simulink model "Simulator_final2019"  (R2019a)
settings: Solver=ode4  StartTime=0  StopTime=500  FixedStep=0.001  RelTol=1e-3
values from neighbouring files (symbols this model uses):
  Control_Matrix = [0   Xde Xdth 0;                   0   0   0    Ydr;                   0   Zde Zdth 0;                   Lda 0   0    Ldr;                   0   Mde Mdth 0;                   Nda 0   0    Ndr]    [Autopilot_Plus_Simulator.m]
  Fg_0 = m * g * [ sin(states_0(8)) ; -cos(states_0(8))*sin(states_0(7)) ; -cos(states_0(8))*cos(states_0(7)) ]    [Autopilot_Plus_Simulator.m]
  g = aircraft_data(52)    [Autopilot_Plus_Simulator.m]
  Ixx = aircraft_data(53)    [Autopilot_Plus_Simulator.m]
  Iyy = aircraft_data(54)    [Autopilot_Plus_Simulator.m]
  Izz = aircraft_data(55)    [Autopilot_Plus_Simulator.m]
  m = aircraft_data(51)    [Autopilot_Plus_Simulator.m]
  Servo = tf(10,[1 10])    [Autopilot_Plus_Simulator.m]
  states_0 = aircraft_data(4:15)    [Autopilot_Plus_Simulator.m]
  States_Matrix = [Xu  0  Xw  0  0  0  0;                  0   Yv 0   Yp 0  Yr 0;                  Zu  0  Zw  0  Zq 0  Zwd;                  0   Lv 0   Lp 0  Lr 0;                  Mu  0  Mw  0  Mq 0  Mwd;                  0   Nv 0   Np 0  Nr 0]    [Autopilot_Plus_Simulator.m]
undefined symbols (not defined in the file or in its folder): Earth, S_0, sigbuilder_block, WGS84
libraries: simulink_extras x14, cstblocks x5, dspsigops x5, aerolibfltsims x2, aerolibtransform2 x1, shared6dof x1, aerolibasang x1, SignalEditorBlockLib x1
settings Model: Creator=Lenovo  LastModifiedBy=Elbohy

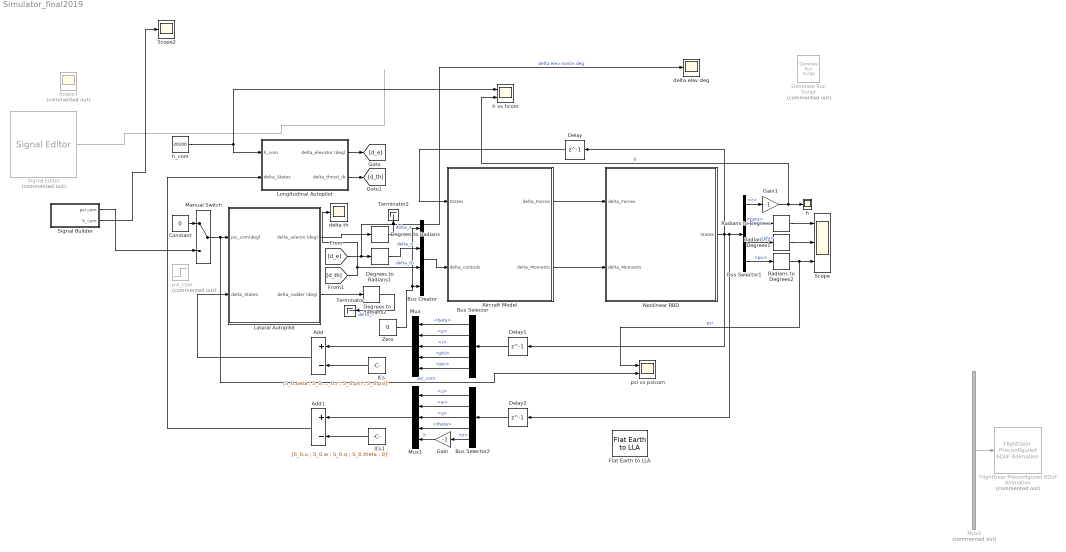
== system Simulator_final2019 ==
  Add : Sum  Inputs=+-
  Add1 : Sum  Inputs=+-
  Aircraft Model : Subsystem
  Bus Creator : BusCreator  Inputs=4
  Bus Selector : BusSelector  OutputSignals=beta,p,r,phi,psi
  Bus Selector1 : BusSelector  OutputSignals=z,beta,phi,psi
  Bus Selector2 : BusSelector  OutputSignals=u,w,q,theta,z
  Constant : Constant  Value=0
  Degrees to Radians : simulink_extras/Transformations/Degrees to Radians
  Degrees to Radians1 : simulink_extras/Transformations/Degrees to Radians
  Degrees to Radians2 : simulink_extras/Transformations/Degrees to Radians
  Delay : Delay  DelayLength=1  InitialCondition=S_0
  Delay1 : Delay  DelayLength=1  InitialCondition=S_0
  Delay2 : Delay  DelayLength=1  InitialCondition=S_0
  Flat Earth to LLA : aerolibtransform2/Flat Earth to LLA  units=Metric (MKS)  ptype=Earth (WGS84)  F=1/298.257223563  R=6378137  LL0=[0 10]  psi=0
  FlightGear Preconfigured 6DoF Animation : aerolibfltsims/FlightGear Preconfigured 6DoF Animation  Commented=on  xFlightGearVersion=v2018.2  DestinationIpAddress=127.0.0.1  DestinationPort=5502  SampleTime=1/30  packetVersion=24
      settings: SourceProductName=Aerospace Blockset
  Gain : Gain  Gain=-1
  Gain1 : Gain  Gain=-1
  Generate Run Script : aerolibfltsims/Generate Run Script  Commented=on  Architecture=Default  dataFlow=Send  GeometryModelName=HL20  AirportId=KSFO  RunwayId=10L  InitialAltitude=7224  InitialHeading=113  OffsetDistance=4.72  OffsetAzimuth=0  InstallScenery=off  DisableShaders=off  OriginAddress=127.0.0.1  DestinationPort=5502  OriginPort=5505  LocalAddress=127.0.0.1  OutputFileName=runfg.bat  FlightGearBaseDirectory=C:\Program Files\FlightGear
  ICs : Constant  Value=[S_0.beta ; S_0.p ; S_0.r ; S_0.phi ; S_0.psi]'
  ICs1 : Constant  Value=[S_0.u ; S_0.w ; S_0.q ; S_0.theta ; 0]'
  Lateral Autopilot : Subsystem
  Longitudinal Autopilot : Subsystem
  Manual Switch : ManualSwitch
  Mux : Mux  Inputs=5
  Mux1 : Mux  Inputs=5
  Mux2 : Mux  Commented=on  Inputs=6
  Nonlinear RBD : Subsystem
  Radians to Degrees : simulink_extras/Transformations/Radians to Degrees
  Radians to Degrees1 : simulink_extras/Transformations/Radians to Degrees
  Radians to Degrees2 : simulink_extras/Transformations/Radians to Degrees
  Scope : Scope  NumInputPorts=3
  Scope2 : Scope
  Scope3 : Scope  Commented=on
  Signal Builder : Subsystem  Tag=STV Subsys  LoadFcn=sigbuilder_block('load');  StartFcn=sigbuilder_block('start');  StopFcn=sigbuilder_block('stop');  ClipboardFcn=sigbuilder_block('clipboard');  mask(Sigbuilder block){tuvar=[0:10]}
      mask help: Simulink:masks:SigbuilderBlock_MD
      mask init:
      | if ~strcmp(get_param(bdroot(gcbh),'SimulationStatus'),'stopped') tuvar = sigbuilder_block('maskInit'); end
      settings: CopyFcn=sigbuilder_block('copy');  DeleteFcn=sigbuilder_block('delete');  ModelCloseFcn=sigbuilder_block('modelClose');  PreSaveFcn=sigbuilder_block('preSave');  PauseFcn=sigbuilder_block('pause');  ContinueFcn=sigbuilder_block('continue');  NameChangeFcn=sigbuilder_block('namechange');  OpenFcn=sigbuilder_block('open',[293.4 123.6 550.8 400.2 ]);  CloseFcn=sigbuilder_block('close');
      mask Display: plot(0, 0, 100, 100,[2, 2, 32, 32, 2], [68, 8, 8, 68, 68],[32, 2], [38, 38], [32, 19, 2],[53, 60, 44], [32, 17, 17, 2],[16, 16, 31, 31]);txt = getActiveGroup(gcbh);text(2, 100, txt,'verticalAlignment', 'top');
  Signal Editor : SignalEditorBlockLib/Signal Editor  Commented=on  FileName=C:\Users\amr ehab\Downloads\final task\scen.mat  ActiveScenario=Scenario  ActiveSignal=psiCommand  IsBus=off  OutputBusObjectStr=Bus: BusObject  SampleTime=0  ZeroCross=off  OutputAfterFinalValue=Holding final value  Unit=inherit  PreserveSignalName=on
      settings: SourceProductName=Simulink
  Terminator : Terminator
  Terminator2 : Terminator
  Zero : Constant  Value=0  OutDataTypeStr=Inherit: Inherit via back propagation
  "delta elav deg " : Scope
  delta th : Scope
  h : Scope
  h vs hcom : Scope  NumInputPorts=2
  h_com : Constant  Value=20100
  psi vs psicom : Scope  NumInputPorts=2
  psi_com : Step  Commented=on  After=360  SampleTime=0
  wires:
  Aircraft Model/2(delta_Moments) -> Nonlinear RBD/2(delta_Moments)
  Aircraft Model/1(delta_Forces) -> Nonlinear RBD/1(delta_Forces)
  Lateral Autopilot/1(delta_aileron (deg)) -> Degrees to Radians/1
  [d_e] -> "delta elav deg "/1, Degrees to Radians1/1  "delta elev nonlin deg"
  Lateral Autopilot/2(delta_rudder (deg)) -> Degrees to Radians2/1
  Degrees to Radians2/1 -> Terminator/1  "delta_r"
  [d_th] -> delta th/1, Bus Creator/3  "delta_th"
  Degrees to Radians1/1 -> Bus Creator/2  "delta_e"
  Degrees to Radians/1 -> Terminator2/1  "delta_a"
  Bus Creator/1 -> Aircraft Model/2(delta_controls)
  Delay/1 -> Aircraft Model/1(States)
  Delay1/1 -> Bus Selector/1
  Bus Selector/1 -> Mux/1  "<beta>"
  Bus Selector/2 -> Mux/2  "<p>"
  Bus Selector/3 -> Mux/3  "<r>"
  Bus Selector/4 -> Mux/4  "<phi>"
  Bus Selector/5 -> Mux/5  "<psi>"
  Mux/1 -> Add/1
  ICs/1 -> Add/2
  Add/1 -> Lateral Autopilot/2(delta_States)
  Bus Selector1/2 -> Radians to Degrees/1  "<beta>"
  Bus Selector1/3 -> Radians to Degrees1/1  "<phi>"
  Bus Selector1/4 -> Radians to Degrees2/1  "<psi>"
  Bus Selector1/1 -> Gain1/1  "<z>"
  Radians to Degrees/1 -> Scope/1
  Radians to Degrees2/1 -> psi vs psicom/1, Scope/3  "psi"
  Radians to Degrees1/1 -> Scope/2
  ICs1/1 -> Add1/2
  Mux1/1 -> Add1/1
  Bus Selector2/2 -> Mux1/2  "<w>"
  Bus Selector2/4 -> Mux1/4  "<theta>"
  Bus Selector2/3 -> Mux1/3  "<q>"
  Delay2/1 -> Bus Selector2/1
  Nonlinear RBD/1(States) -> Delay1/1, Delay2/1, Bus Selector1/1, Delay/1
  Bus Selector2/1 -> Mux1/1  "<u>"
  Longitudinal Autopilot/1(delta_elevator (deg)) -> [d_e]
  Longitudinal Autopilot/2("delta_thrust_ib ") -> [d_th]
  Bus Selector2/5 -> Gain/1  "<z>"
  Add1/1 -> Longitudinal Autopilot/2(delta_States)
  Gain/1 -> Mux1/5  "h"
  Manual Switch/1 -> psi vs psicom/2, Lateral Autopilot/1(psi_com(deg))  "psi_com"
  Constant/1 -> Manual Switch/1
  Gain1/1 -> h vs hcom/2, h/1  "h"
  ? -> Scope3/1
  Signal Editor/1 -> ?
  Mux2/1 -> FlightGear Preconfigured 6DoF Animation/1
  ? -> Mux2/1
  ? -> Mux2/2
  ? -> Mux2/3
  ? -> Mux2/4
  ? -> Mux2/5
  ? -> Mux2/6
  Signal Builder/2(h_com) -> Scope2/1
  Signal Builder/1(psi com) -> Manual Switch/2
  h_com/1 -> Longitudinal Autopilot/1(h_com), h vs hcom/1
  Zero/1 -> Bus Creator/1, Bus Creator/4

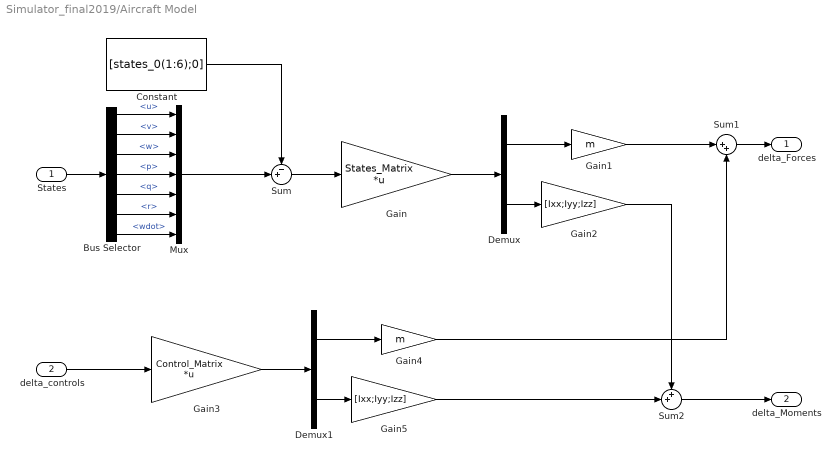
== system Simulator_final2019/Aircraft Model ==
  States : Inport
  delta_controls : Inport  Port=2
  Bus Selector : BusSelector  OutputSignals=u,v,w,p,q,r,wdot
  Constant : Constant  Value=[states_0(1:6);0]
  Demux : Demux  Outputs=2
  Demux1 : Demux  Outputs=2
  Gain : Gain  Gain=States_Matrix  Multiplication=Matrix(K*u)
  Gain1 : Gain  Gain=m
  Gain2 : Gain  Gain=[Ixx;Iyy;Izz]
  Gain3 : Gain  Gain=Control_Matrix  Multiplication=Matrix(K*u)
  Gain4 : Gain  Gain=m
  Gain5 : Gain  Gain=[Ixx;Iyy;Izz]
  Mux : Mux  Inputs=7
  Sum : Sum  Inputs=-+|
  Sum1 : Sum  Inputs=|++
  Sum2 : Sum  Inputs=++|
  delta_Forces : Outport  VectorParamsAs1DForOutWhenUnconnected=on
  delta_Moments : Outport  Port=2  VectorParamsAs1DForOutWhenUnconnected=on
  wires:
  Gain5/1 -> Sum2/2
  Gain1/1 -> Sum1/1
  Demux/2 -> Gain2/1
  Constant/1 -> Sum/1
  Gain/1 -> Demux/1
  Sum/1 -> Gain/1
  Mux/1 -> Sum/2
  Gain3/1 -> Demux1/1
  Gain4/1 -> Sum1/2
  Demux/1 -> Gain1/1
  Demux1/1 -> Gain4/1
  Demux1/2 -> Gain5/1
  Gain2/1 -> Sum2/1
  Sum1/1 -> delta_Forces/1
  Sum2/1 -> delta_Moments/1
  Bus Selector/1 -> Mux/1  "<u>"
  Bus Selector/2 -> Mux/2  "<v>"
  Bus Selector/3 -> Mux/3  "<w>"
  Bus Selector/4 -> Mux/4  "<p>"
  Bus Selector/5 -> Mux/5  "<q>"
  Bus Selector/6 -> Mux/6  "<r>"
  Bus Selector/7 -> Mux/7  "<wdot>"
  States/1 -> Bus Selector/1
  delta_controls/1 -> Gain3/1

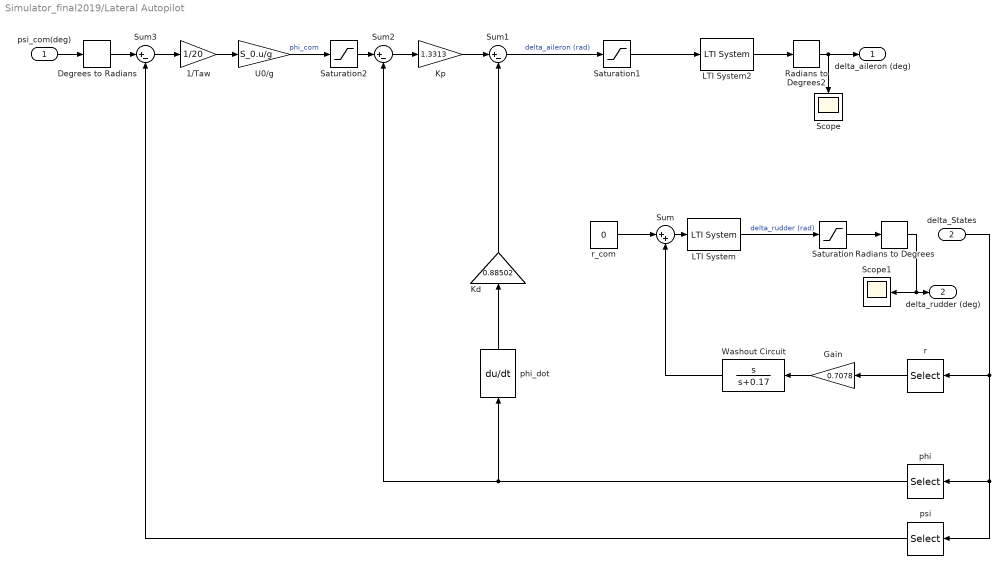
== system Simulator_final2019/Lateral Autopilot ==
  psi_com(deg) : Inport
  delta_States : Inport  Port=2
  1/Taw : Gain  Gain=1/20
  Degrees to Radians : simulink_extras/Transformations/Degrees to Radians
  Gain : Gain  Gain=0.7078
  Kd : Gain  Gain=0.88502
  Kp : Gain  Gain=1.3313
  LTI System : cstblocks/LTI System  sys=servo  IC=[]
  LTI System2 : cstblocks/LTI System  sys=servo  IC=[]
  Radians to Degrees : simulink_extras/Transformations/Radians to Degrees
  Radians to Degrees2 : simulink_extras/Transformations/Radians to Degrees
  Saturation : Saturate  UpperLimit=15*pi/180  LowerLimit=-15*pi/180
  Saturation1 : Saturate  UpperLimit=50*pi/180  LowerLimit=-50*pi/180
  Saturation2 : Saturate  UpperLimit=30*pi/180  LowerLimit=-30*pi/180
  Scope : Scope
  Scope1 : Scope
  Sum : Sum  Inputs=|++
  Sum1 : Sum  Inputs=|+-
  Sum2 : Sum  Inputs=|+-
  Sum3 : Sum  Inputs=|+-
  U0/g : Gain  Gain=S_0.u/g
  Washout Circuit : TransferFcn  Numerator=[1 0]  Denominator=[1 0.17]
  phi : Selector  InputPortWidth=5  IndexOptions=Index vector (dialog)  Indices=[4]  OutputSizes=1
  phi_dot : Derivative
  psi : Selector  InputPortWidth=5  IndexOptions=Index vector (dialog)  Indices=[5]  OutputSizes=1
  r : Selector  InputPortWidth=5  IndexOptions=Index vector (dialog)  Indices=[3]  OutputSizes=1
  r_com : Constant  Value=0
  delta_aileron (deg) : Outport  VectorParamsAs1DForOutWhenUnconnected=on
  delta_rudder (deg) : Outport  Port=2  VectorParamsAs1DForOutWhenUnconnected=on
  wires:
  LTI System2/1 -> Radians to Degrees2/1
  1/Taw/1 -> U0/g/1
  Kp/1 -> Sum1/1
  Radians to Degrees2/1 -> delta_aileron (deg)/1, Scope/1
  Sum1/1 -> Saturation1/1  "delta_aileron (rad)"
  delta_States/1 -> phi/1, psi/1, r/1
  Saturation2/1 -> Sum2/1
  Radians to Degrees/1 -> Scope1/1, delta_rudder (deg)/1
  Kd/1 -> Sum1/2
  Sum2/1 -> Kp/1
  psi/1 -> Sum3/2
  Saturation1/1 -> LTI System2/1
  LTI System/1 -> Saturation/1  "delta_rudder (rad)"
  phi/1 -> Sum2/2, phi_dot/1
  Gain/1 -> Washout Circuit/1
  Sum3/1 -> 1/Taw/1
  Washout Circuit/1 -> Sum/2
  r_com/1 -> Sum/1
  r/1 -> Gain/1
  Degrees to Radians/1 -> Sum3/1
  U0/g/1 -> Saturation2/1  "phi_com"
  Saturation/1 -> Radians to Degrees/1
  phi_dot/1 -> Kd/1
  Sum/1 -> LTI System/1
  psi_com(deg)/1 -> Degrees to Radians/1

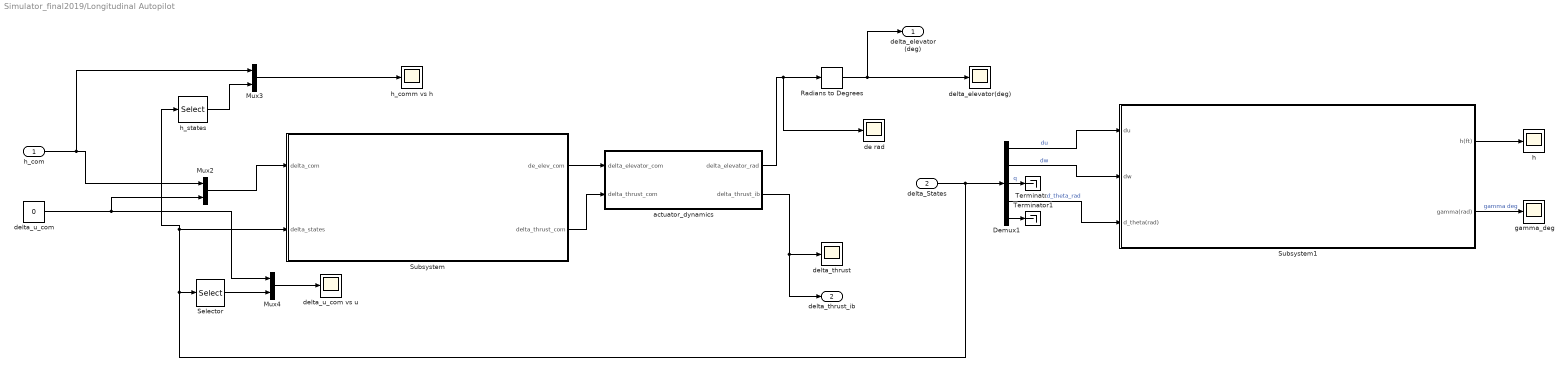
== system Simulator_final2019/Longitudinal Autopilot ==
  h_com : Inport
  delta_States : Inport  Port=2
  Demux1 : Demux  Outputs=5
  Mux2 : Mux  Inputs=2
  Mux3 : Mux  Inputs=2
  Mux4 : Mux  Inputs=2
  Radians to Degrees : simulink_extras/Transformations/Radians to Degrees
  Selector : Selector  InputPortWidth=5  IndexOptions=Index vector (dialog)  Indices=[1]  OutputSizes=1
  Subsystem : Subsystem
  Subsystem1 : Subsystem
  Terminator : Terminator
  Terminator1 : Terminator
  "actuator_dynamics " : Subsystem
  de rad : Scope
  delta_elevator(deg) : Scope
  delta_thrust : Scope
  delta_u_com : Constant  Value=0
  "delta_u_com vs u " : Scope
  gamma_deg : Scope
  h : Scope
  h_comm vs h : Scope
  h_states : Selector  InputPortWidth=5  IndexOptions=Index vector (dialog)  Indices=[5]  OutputSizes=1
  delta_elevator (deg) : Outport  VectorParamsAs1DForOutWhenUnconnected=on
  "delta_thrust_ib " : Outport  Port=2  VectorParamsAs1DForOutWhenUnconnected=on
  wires:
  h_com/1 -> Mux3/1, Mux2/1
  Mux2/1 -> Subsystem/1(delta_com)
  Radians to Degrees/1 -> delta_elevator (deg)/1, delta_elevator(deg)/1
  Subsystem1/1("h(ft) ") -> h/1
  Subsystem/2(delta_thrust_com) -> "actuator_dynamics "/2("delta_thrust_com ")
  delta_States/1 -> Selector/1, h_states/1, Subsystem/2("delta_states "), Demux1/1
  delta_u_com/1 -> Mux4/1, Mux2/2
  Selector/1 -> Mux4/2
  Demux1/1 -> Subsystem1/1("du ")  "du"
  Subsystem1/2(gamma(rad)) -> gamma_deg/1  "gamma deg"
  Demux1/4 -> Subsystem1/3(d_theta(rad))  "d_theta_rad"
  "actuator_dynamics "/2("delta_thrust_ib ") -> "delta_thrust_ib "/1, delta_thrust/1
  h_states/1 -> Mux3/2
  Demux1/2 -> Subsystem1/2(dw)  "dw"
  Mux3/1 -> h_comm vs h/1
  "actuator_dynamics "/1(delta_elevator_rad) -> de rad/1, Radians to Degrees/1
  Subsystem/1(de_elev_com) -> "actuator_dynamics "/1("delta_elevator_com ")
  Mux4/1 -> "delta_u_com vs u "/1
  Demux1/3 -> Terminator/1  "q"
  Demux1/5 -> Terminator1/1

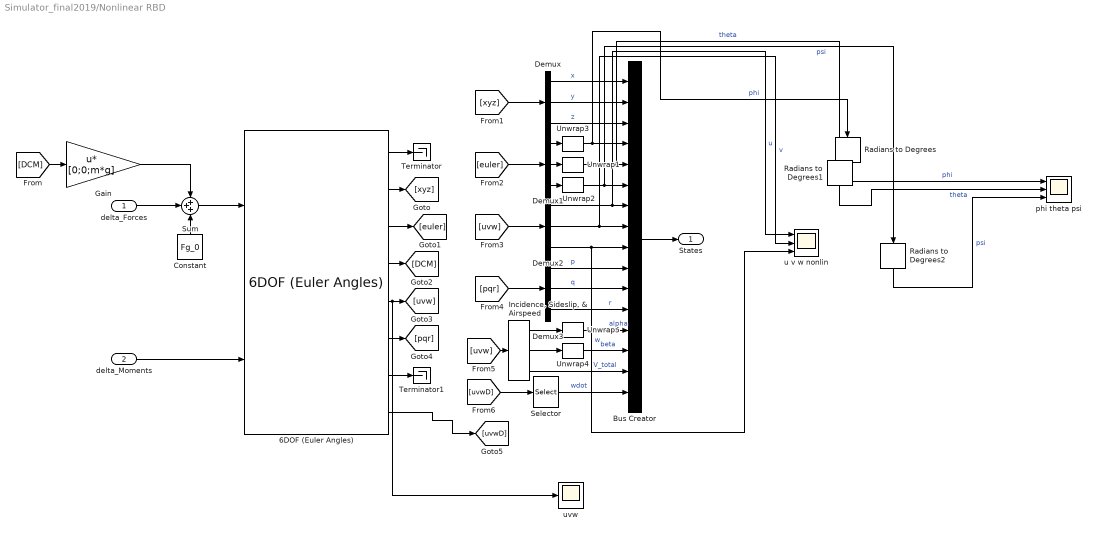
== system Simulator_final2019/Nonlinear RBD ==
  delta_Forces : Inport
  delta_Moments : Inport  Port=2
  6DOF (Euler Angles) : shared6dof/6DOF (Euler Angles)  units=English (Velocity in ft/s)  mtype=Fixed  rep=Euler Angles  xme_0=states_0(10:12)  Vm_0=states_0(1:3)  eul_0=states_0(7:9)  pm_0=states_0(4:6)  mass_0=m  mass_e=0.5  mass_f=2.0  inertia=I  inertia_e=eye(3)  inertia_f=2*eye(3)  k_quat=1.0  vre_flag=on  abi_flag=off  aMode=0  xme_statename=''  Vm_statename=''  eul_statename=''  quat_statename=''  pm_statename=''  mass_statename=''
      settings: SourceProductBaseCode=AE
  Bus Creator : BusCreator  Inputs=16
  Constant : Constant  Value=Fg_0
  Demux{,1..3} (4 alike) : Demux  Outputs=3
  Gain : Gain  Gain=[0;0;m*g]  Multiplication=Matrix(u*K)
  "Incidence, Sideslip, & Airspeed" : aerolibasang/Incidence, Sideslip, & Airspeed
      settings: SourceProductName=Aerospace Blockset
  Radians to Degrees : simulink_extras/Transformations/Radians to Degrees
  Radians to Degrees1 : simulink_extras/Transformations/Radians to Degrees
  Radians to Degrees2 : simulink_extras/Transformations/Radians to Degrees
  Selector : Selector  InputPortWidth=3  IndexOptions=Index vector (dialog)  Indices=[3]  OutputSizes=1
  Sum : Sum  Inputs=+++
  Terminator : Terminator
  Terminator1 : Terminator
  Unwrap{1..5} (5 alike) : dspsigops/Unwrap  tol=pi  InputProcessing=Columns as channels (frame based)  running=off
  phi theta psi : Scope  NumInputPorts=3
  u v w nonlin : Scope  NumInputPorts=3
  "uvw " : Scope
  States : Outport  VectorParamsAs1DForOutWhenUnconnected=on
  wires:
  Demux2/1 -> u v w nonlin/1, Bus Creator/7  "u"
  Selector/1 -> Bus Creator/16  "wdot"
  Demux/1 -> Bus Creator/1  "x"
  Demux1/1 -> Unwrap3/1
  Demux3/3 -> Bus Creator/12  "r"
  Demux3/2 -> Bus Creator/11  "q"
  [xyz] -> Demux/1
  Demux1/2 -> Unwrap1/1
  Demux/3 -> Bus Creator/3  "z"
  [pqr] -> Demux3/1
  [uvw] -> Demux2/1
  [uvw] -> "Incidence, Sideslip, & Airspeed"/1
  Gain/1 -> Sum/1
  6DOF (Euler Angles)/5 -> "uvw "/1, [uvw]
  "Incidence, Sideslip, & Airspeed"/3 -> Bus Creator/15  "V_total"
  6DOF (Euler Angles)/3 -> [euler]
  6DOF (Euler Angles)/4 -> [DCM]
  Demux2/2 -> u v w nonlin/2, Bus Creator/8  "v"
  Demux2/3 -> u v w nonlin/3, Bus Creator/9  "w"
  6DOF (Euler Angles)/6 -> [pqr]
  Demux/2 -> Bus Creator/2  "y"
  [uvwD] -> Selector/1
  6DOF (Euler Angles)/1 -> Terminator/1
  Sum/1 -> 6DOF (Euler Angles)/1
  6DOF (Euler Angles)/8 -> [uvwD]
  [euler] -> Demux1/1
  [DCM] -> Gain/1
  6DOF (Euler Angles)/7 -> Terminator1/1
  Demux3/1 -> Bus Creator/10  "p"
  Constant/1 -> Sum/3
  6DOF (Euler Angles)/2 -> [xyz]
  delta_Forces/1 -> Sum/2
  delta_Moments/1 -> 6DOF (Euler Angles)/2
  Bus Creator/1 -> States/1
  Unwrap1/1 -> Radians to Degrees1/1, Bus Creator/5  "theta"
  Demux1/3 -> Unwrap2/1
  Unwrap3/1 -> Radians to Degrees/1, Bus Creator/4  "phi"
  Unwrap2/1 -> Bus Creator/6, Radians to Degrees2/1  "psi"
  "Incidence, Sideslip, & Airspeed"/2 -> Unwrap4/1
  Unwrap5/1 -> Bus Creator/13  "alpha"
  Unwrap4/1 -> Bus Creator/14  "beta"
  "Incidence, Sideslip, & Airspeed"/1 -> Unwrap5/1
  Radians to Degrees/1 -> phi theta psi/1  "phi"
  Radians to Degrees1/1 -> phi theta psi/2  "theta"
  Radians to Degrees2/1 -> phi theta psi/3  "psi"

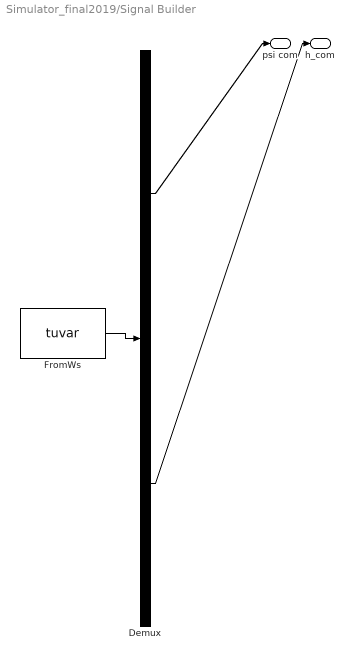
== system Simulator_final2019/Signal Builder ==
  Demux : Demux  Tag=STV Demux  Outputs=2
  FromWs : FromWorkspace  Tag=STV FromWs  VariableName=tuvar  SampleTime=0
      SigBuilderData=|
      | common.afterFinalStr = 'Extrapolate'
      | common.sampleTime = 0
      | dataSet.timeRange = [0 1800]
      | dataSet.name = 'Group 1'
      | sbobj.Groups.Name = 'Group 1'
      | sbobj.Groups.Signals(1).Name = 'psi com'
      | sbobj.Groups.Signals(1).XData = [0 720 720 1080 1080 1800]
      | sbobj.Groups.Signals(1).YData = [0 0 360 360 390 390]
      | sbobj.Groups.Signals(2).Name = 'h_com'
      | sbobj.Groups.Signals(2).XData = [0 600 1080 1080 1200 1800]
      | sbobj.Groups.Signals(2).YData = [20000 30000 30000 30100 30100 20000]
      | sbobj.Groups.TimeRange = [0 1800]
  psi com : Outport  Tag=STV Outport
  h_com : Outport  Tag=STV Outport  Port=2
  wires:
  FromWs/1 -> Demux/1
  Demux/1 -> psi com/1
  Demux/2 -> h_com/1

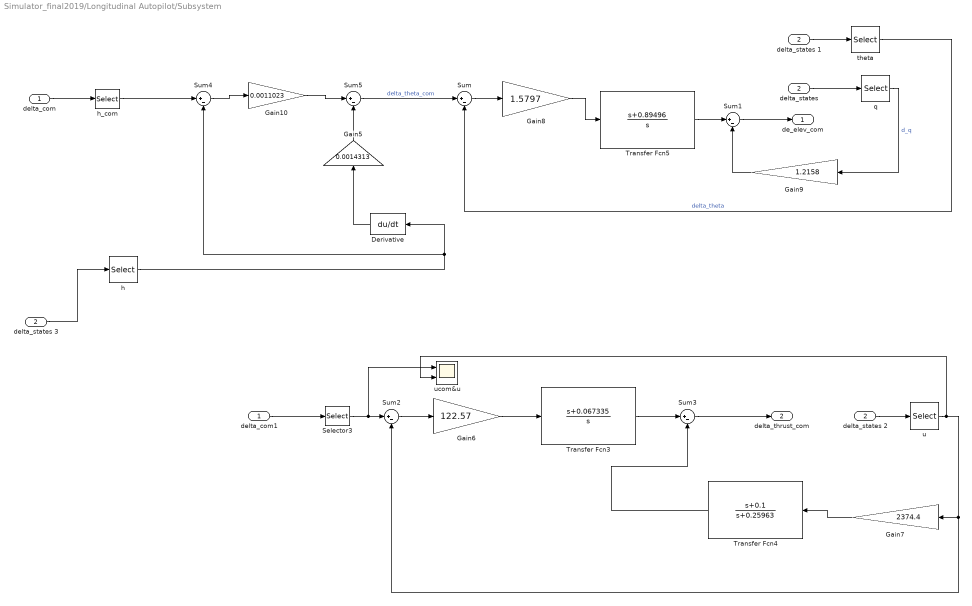
== system Simulator_final2019/Longitudinal Autopilot/Subsystem ==
  delta_com : Inport
  "delta_states " : Inport  Port=2
  Derivative : Derivative
  Gain10 : Gain  Gain=0.0011023
  Gain5 : Gain  Gain=0.0014313
  Gain6 : Gain  Gain=122.57
  Gain7 : Gain  Gain=2374.4
  Gain8 : Gain  Gain=1.5797
  Gain9 : Gain  Gain=1.2158
  Selector3 : Selector  InputPortWidth=2  IndexOptions=Index vector (dialog)  Indices=[2]  OutputSizes=1
  Sum{,1..5} (6 alike) : Sum  Inputs=|+-
  Transfer Fcn3 : TransferFcn  Numerator=[1 0.067335]  Denominator=[1 0]
  Transfer Fcn4 : TransferFcn  Numerator=[1 0.1]  Denominator=[1 0.25963]
  Transfer Fcn5 : TransferFcn  Numerator=[1 0.89496]  Denominator=[1 0]
  delta_com1 : InportShadow
  delta_states 1 : InportShadow  Port=2
  delta_states 2 : InportShadow  Port=2
  delta_states 3 : InportShadow  Port=2
  h : Selector  InputPortWidth=5  IndexOptions=Index vector (dialog)  Indices=[5]  OutputSizes=1
  h_com : Selector  InputPortWidth=2  IndexOptions=Index vector (dialog)  Indices=[1]  OutputSizes=1
  "q " : Selector  InputPortWidth=5  IndexOptions=Index vector (dialog)  Indices=[3]  OutputSizes=1
  "theta " : Selector  InputPortWidth=5  IndexOptions=Index vector (dialog)  Indices=[4]  OutputSizes=1
  u : Selector  InputPortWidth=5  IndexOptions=Index vector (dialog)  Indices=[1]  OutputSizes=1
  ucom&u : Scope  NumInputPorts=2
  de_elev_com : Outport
  delta_thrust_com : Outport  Port=2
  wires:
  Gain10/1 -> Sum5/1
  Gain5/1 -> Sum5/2
  Gain8/1 -> Transfer Fcn5/1
  delta_com/1 -> h_com/1
  Sum/1 -> Gain8/1
  delta_states 3/1 -> h/1
  h/1 -> Derivative/1, Sum4/2
  delta_com1/1 -> Selector3/1
  delta_states 2/1 -> u/1
  Gain7/1 -> Transfer Fcn4/1
  "delta_states "/1 -> "q "/1
  "q "/1 -> Gain9/1  "d_q"
  delta_states 1/1 -> "theta "/1
  Gain6/1 -> Transfer Fcn3/1
  Sum1/1 -> de_elev_com/1
  Transfer Fcn4/1 -> Sum3/2
  Transfer Fcn5/1 -> Sum1/1
  Sum5/1 -> Sum/1  "delta_theta_com"
  Selector3/1 -> ucom&u/1, Sum2/1
  Gain9/1 -> Sum1/2
  Sum4/1 -> Gain10/1
  "theta "/1 -> Sum/2  "delta_theta"
  Transfer Fcn3/1 -> Sum3/1
  u/1 -> ucom&u/2, Gain7/1, Sum2/2
  Sum2/1 -> Gain6/1
  h_com/1 -> Sum4/1
  Sum3/1 -> delta_thrust_com/1
  Derivative/1 -> Gain5/1

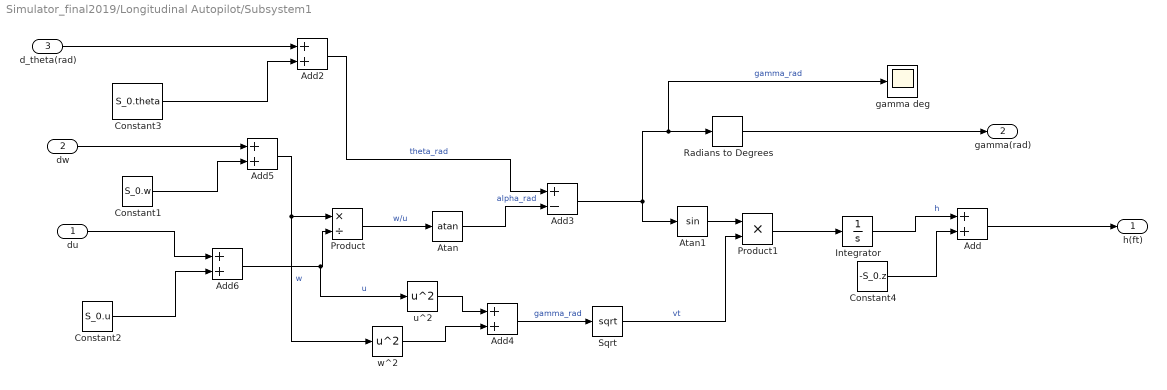
== system Simulator_final2019/Longitudinal Autopilot/Subsystem1 ==
  "du " : Inport
  dw : Inport  Port=2
  d_theta(rad) : Inport  Port=3
  Add{,2,4..6} (5 alike) : Sum
  Add3 : Sum  Inputs=+-
  Atan : Trigonometry  Operator=atan
  Atan1 : Trigonometry
  Constant1 : Constant  Value=S_0.w
  Constant2 : Constant  Value=S_0.u
  Constant3 : Constant  Value=S_0.theta
  Constant4 : Constant  Value=-S_0.z
  Integrator : Integrator
  Product : Product  Inputs=*/
  Product1 : Product
  Radians to Degrees : simulink_extras/Transformations/Radians to Degrees
  Sqrt : Sqrt  SaturateOnIntegerOverflow=on
  gamma deg : Scope
  u^2 : Math  Operator=square  SaturateOnIntegerOverflow=on
  w^2 : Math  Operator=square  SaturateOnIntegerOverflow=on
  "h(ft) " : Outport
  gamma(rad) : Outport  Port=2
  wires:
  Product1/1 -> Integrator/1
  Constant4/1 -> Add/2
  Radians to Degrees/1 -> gamma(rad)/1
  Integrator/1 -> Add/1  "h"
  dw/1 -> Add5/1
  d_theta(rad)/1 -> Add2/1
  Atan/1 -> Add3/2  "alpha_rad"
  Constant2/1 -> Add6/2
  Constant1/1 -> Add5/2
  Add4/1 -> Sqrt/1  "gamma_rad"
  u^2/1 -> Add4/1
  w^2/1 -> Add4/2
  "du "/1 -> Add6/1
  Atan1/1 -> Product1/1
  Sqrt/1 -> Product1/2  "vt"
  Constant3/1 -> Add2/2
  Add5/1 -> Product/1, w^2/1  "w"
  Add2/1 -> Add3/1  "theta_rad"
  Product/1 -> Atan/1  "w/u"
  Add6/1 -> u^2/1, Product/2  "u"
  Add3/1 -> Atan1/1, gamma deg/1, Radians to Degrees/1  "gamma_rad"
  Add/1 -> "h(ft) "/1

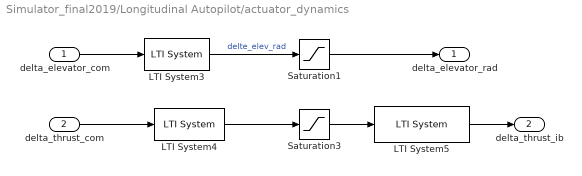
== system Simulator_final2019/Longitudinal Autopilot/actuator_dynamics  ==
  "delta_elevator_com " : Inport
  "delta_thrust_com " : Inport  Port=2
  LTI System3 : cstblocks/LTI System  sys=-Servo  IC=[]
  LTI System4 : cstblocks/LTI System  sys=Servo  IC=[]
  LTI System5 : cstblocks/LTI System  sys=Engine_Time_lag  IC=[]
  Saturation1 : Saturate  UpperLimit=25*pi/180  LowerLimit=-25*pi/180
  Saturation3 : Saturate  UpperLimit=57000  LowerLimit=-150000
  delta_elevator_rad : Outport
  "delta_thrust_ib " : Outport  Port=2
  wires:
  LTI System3/1 -> Saturation1/1  "delte_elev_rad"
  LTI System5/1 -> "delta_thrust_ib "/1
  Saturation1/1 -> delta_elevator_rad/1
  LTI System4/1 -> Saturation3/1
  Saturation3/1 -> LTI System5/1
  "delta_thrust_com "/1 -> LTI System4/1
  "delta_elevator_com "/1 -> LTI System3/1
